simulink model "test05"  (R2017a)
settings: Solver=FixedStepAuto  StartTime=0.0  StopTime=4.95  RelTol=1e-3
libraries: commchan3 x1
settings Model: Creator=58406  LastModifiedBy=58406

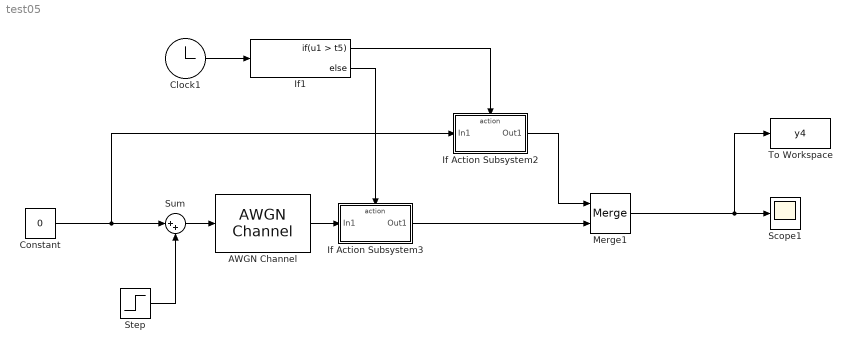
== system test05 ==
  AWGN Channel : commchan3/AWGN Channel  InputProcessing=Columns as channels (frame based)  seed=seed  noiseMode="Signal to noise ratio  (SNR)"  EbNodB=36  EsNodB=10  SNRdB=36  bitsPerSym=1  Ps=1  Tsym=1  variance=1
  Clock1 : Clock
  Constant : Constant  Value=0
  If Action Subsystem2 : Subsystem  TreatAsAtomicUnit=on
  If Action Subsystem3 : Subsystem  TreatAsAtomicUnit=on
  If1 : If  IfExpression=u1 > t5
  Merge1 : Merge
  Scope1 : Scope
  Step : Step  Time=0  SampleTime=0.05
  Sum : Sum  Inputs=|++
  To Workspace : ToWorkspace  VariableName=y4  SampleTime=-1
      settings: Save2DSignal=2-D array (concatenate along first dimension)
  wires:
  If Action Subsystem3/1(Out1) -> Merge1/2
  If1/2 -> If Action Subsystem3/Action
  Constant/1 -> Sum/1, If Action Subsystem2/1(In1)
  Clock1/1 -> If1/1
  If1/1 -> If Action Subsystem2/Action
  Merge1/1 -> To Workspace/1, Scope1/1
  If Action Subsystem2/1(Out1) -> Merge1/1
  Step/1 -> Sum/2
  Sum/1 -> AWGN Channel/1
  AWGN Channel/1 -> If Action Subsystem3/1(In1)

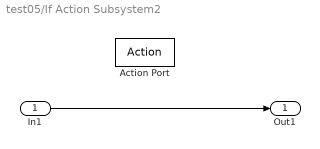
== system test05/If Action Subsystem2 ==
  In1 : Inport
  Action Port : ActionPort  ActionType=then
  Out1 : Outport
  wires:
  In1/1 -> Out1/1

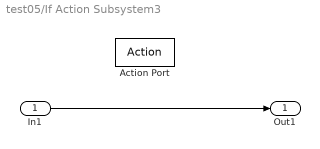
== system test05/If Action Subsystem3 ==
  In1 : Inport
  Action Port : ActionPort  ActionType=else
  Out1 : Outport
  wires:
  In1/1 -> Out1/1
